simulink model "tests_feedforward_shapers"  (R2015b)
settings: Solver=FixedStepAuto  StartTime=0.0  StopTime=10.0  FixedStep=0.001  RelTol=1e-3
undefined symbols (not defined in the file): a, tau, tau_sub
libraries: cstblocks x3
settings Model: Creator=dave  LastModifiedBy=dave

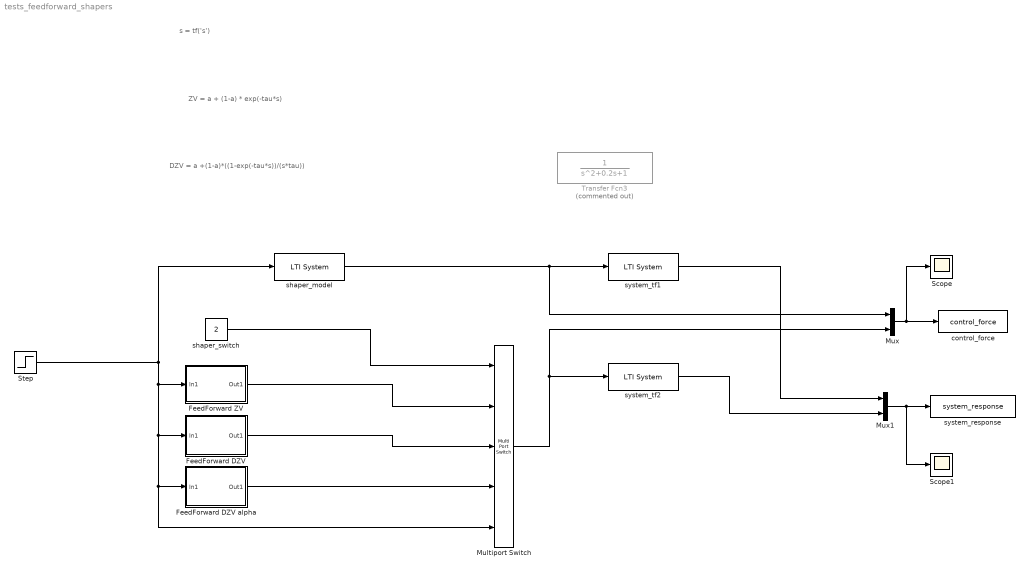
== system tests_feedforward_shapers ==
  note: s = tf('s')
  note: ZV = a + (1-a) * exp(-tau*s)
  note: DZV = a +(1-a)*((1-exp(-tau*s))/(s*tau))
  FeedForward DZV : Subsystem
  FeedForward DZV alpha : Subsystem
  FeedForward ZV : Subsystem
  Multiport Switch : MultiPortSwitch  Inputs=4
  Mux : Mux  Inputs=2
  Mux1 : Mux  Inputs=2
  Scope : Scope
  Scope1 : Scope
  Step : Step  SampleTime=0
  Transfer Fcn3 : TransferFcn  Commented=on  Denominator=[1 0.2 1]
  control_force : ToWorkspace  VariableName=control_force  SaveFormat=Timeseries  SampleTime=-1
  shaper_model : cstblocks/LTI System  sys=shaper_model  IC=[]
  shaper_switch : Constant  Value=2
  system_response : ToWorkspace  VariableName=system_response  SaveFormat=Timeseries  SampleTime=-1
  system_tf1 : cstblocks/LTI System  sys=system_tf  IC=[]
  system_tf2 : cstblocks/LTI System  sys=system_tf  IC=[]
  wires:
  Step/1 -> Multiport Switch/5, FeedForward DZV alpha/1(In1), FeedForward DZV/1(In1), FeedForward ZV/1(In1), shaper_model/1
  Multiport Switch/1 -> system_tf2/1, Mux/2
  FeedForward DZV/1(Out1) -> Multiport Switch/3
  shaper_switch/1 -> Multiport Switch/1
  FeedForward ZV/1(Out1) -> Multiport Switch/2
  FeedForward DZV alpha/1(Out1) -> Multiport Switch/4
  Mux/1 -> Scope/1, control_force/1
  Mux1/1 -> Scope1/1, system_response/1
  system_tf1/1 -> Mux1/1
  shaper_model/1 -> system_tf1/1, Mux/1
  system_tf2/1 -> Mux1/2

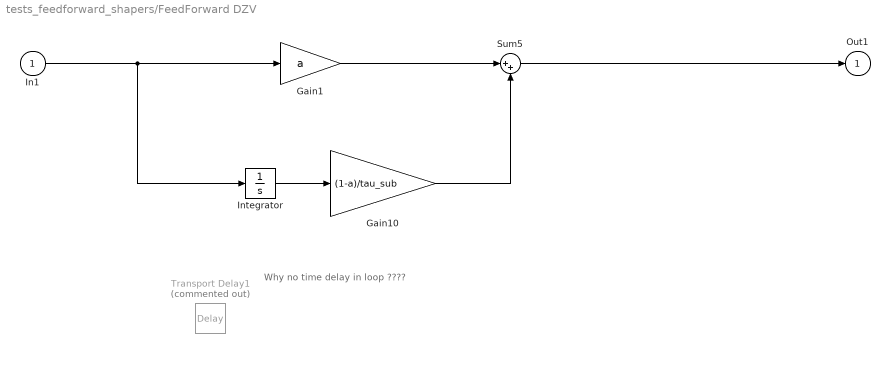
== system tests_feedforward_shapers/FeedForward DZV ==
  note: Why no time delay in loop ????
  In1 : Inport
  Gain1 : Gain  Gain=a
  Gain10 : Gain  Gain=(1-a)/tau_sub
  Integrator : Integrator  LimitOutput=on  UpperSaturationLimit=tau_sub  LowerSaturationLimit=0
  Sum5 : Sum  Inputs=|++
  Transport Delay1 : TransportDelay  Commented=on  DelayTime=tau
  Out1 : Outport
  wires:
  Sum5/1 -> Out1/1
  Integrator/1 -> Gain10/1
  Gain10/1 -> Sum5/2
  Gain1/1 -> Sum5/1
  In1/1 -> Integrator/1, Gain1/1

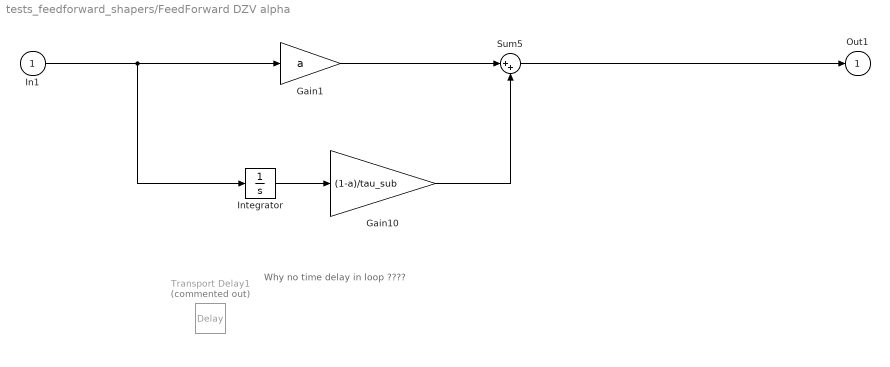
== system tests_feedforward_shapers/FeedForward DZV alpha ==
  note: Why no time delay in loop ????
  In1 : Inport
  Gain1 : Gain  Gain=a
  Gain10 : Gain  Gain=(1-a)/tau_sub
  Integrator : Integrator  LimitOutput=on  UpperSaturationLimit=tau_sub  LowerSaturationLimit=0
  Sum5 : Sum  Inputs=|++
  Transport Delay1 : TransportDelay  Commented=on  DelayTime=tau
  Out1 : Outport
  wires:
  In1/1 -> Gain1/1, Integrator/1
  Gain1/1 -> Sum5/1
  Gain10/1 -> Sum5/2
  Integrator/1 -> Gain10/1
  Sum5/1 -> Out1/1

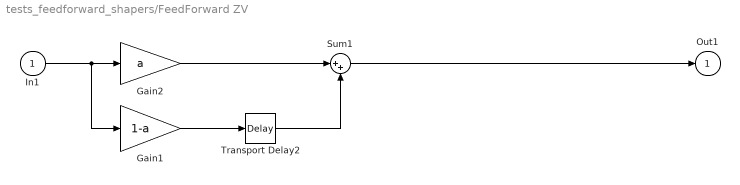
== system tests_feedforward_shapers/FeedForward ZV ==
  In1 : Inport
  Gain1 : Gain  Gain=1-a
  Gain2 : Gain  Gain=a
  Sum1 : Sum  Inputs=|++
  Transport Delay2 : TransportDelay  DelayTime=tau_sub  BufferSize=10000
  Out1 : Outport
  wires:
  Gain1/1 -> Transport Delay2/1
  In1/1 -> Gain1/1, Gain2/1
  Sum1/1 -> Out1/1
  Gain2/1 -> Sum1/1
  Transport Delay2/1 -> Sum1/2
